simulink model "bldc_with_svpwm"  (R2022a)
settings: Solver=FixedStepDiscrete  StartTime=0.0  StopTime=1  RelTol=1e-3
undefined symbols (not defined in the file): Ts, Vdc
libraries: simulink x5, slpidlib x3, spsDCVoltageSourceLib x1, spsPermanentMagnetSynchronousMachineLib x1, spsUniversalBridgeLib x1, spspowerguiLib x1
(part 1 of 2)
settings Model: Creator=XieXW  LastModifiedBy=XieXW

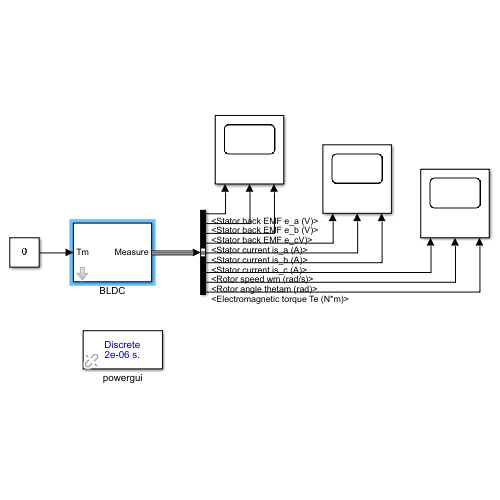
[thumbnail: Simulink's stored preview of the top-level diagram]
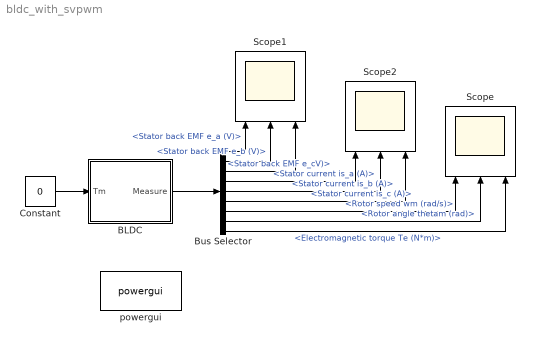
== system bldc_with_svpwm ==
  BLDC : Subsystem  mask{Va=0, Vb=0, Vc=0, t0=0}
      mask prompts: Va "A相电压"; Vb "B相电压"; Vc "C相电压"; t0 "初始角度t0"
      mask DialogControl ParameterGroupVar Prompt: 参数
  Bus Selector : BusSelector  OutputSignals=Stator back EMF e_a (V),Stator back EMF e_b (V),Stator back EMF e_cV),Stator current is_a (A),Stator current is_b (A),Stator current is_c (A),Rotor speed wm (rad/s),Rotor angle thetam (rad),Electromagnetic torque Te (N*m)
  Constant : Constant  Value=0
  Scope : Scope  NumInputPorts=3
  Scope1 : Scope  NumInputPorts=3
  Scope2 : Scope  NumInputPorts=3
  powergui : spspowerguiLib/powergui  Priority=1  SimulationMode=Discrete  SampleTime=2e-6  frequency=60  Iterations=50  frequencyindice=0  Pbase=100e6  ErrMax=1e-4  UnitsV=kV  UnitsW=MW  buscounter=0  FunctionMessages=off  echomessages=off  EnableUseOfTLC=off  CurrentSourceSwitches=off  DisableSnubberDevices=off  DisableRonSwitches=off  DisableVfSwitches=off  DisplayEquations=off  AutomaticDiscreteSolvers=off  SolverType=Tustin/Backward Euler (TBE)  Interpol=off  ExternalGateDelay=off  methode=off  Ts=100  x0status=blocks  SPID=on  SwTol=0  HookPort=off  NonlinearTolerance=1e-4  nMaxIteration=100  ContinueOnMaxIteration=off  RestoreLinks=warning  ResistiveCurrentMeasurement=off  Frange=[0:2:500]  Ylog=off  Xlog=on  ShowGrid=off  save=off  variable=ZData  structure=0  ZoomFFT=off  StartTime=0.0  cycles=1  DisplayStyle=1  fundamental=60  FreqAxis=off  MaxFrequency=1000  frequencyindicesteady=1  RmsSteady=1  display=off
  wires:
  BLDC/1(Measure) -> Bus Selector/1
  Constant/1 -> BLDC/1(Tm)
  Bus Selector/7 -> Scope/1  "<Rotor speed wm (rad/s)>"
  Bus Selector/8 -> Scope/2  "<Rotor angle thetam (rad)>"
  Bus Selector/9 -> Scope/3  "<Electromagnetic torque Te (N*m)>"
  Bus Selector/1 -> Scope1/1  "<Stator back EMF e_a (V)>"
  Bus Selector/2 -> Scope1/2  "<Stator back EMF e_b (V)>"
  Bus Selector/3 -> Scope1/3  "<Stator back EMF e_cV)>"
  Bus Selector/4 -> Scope2/1  "<Stator current is_a (A)>"
  Bus Selector/5 -> Scope2/2  "<Stator current is_b (A)>"
  Bus Selector/6 -> Scope2/3  "<Stator current is_c (A)>"

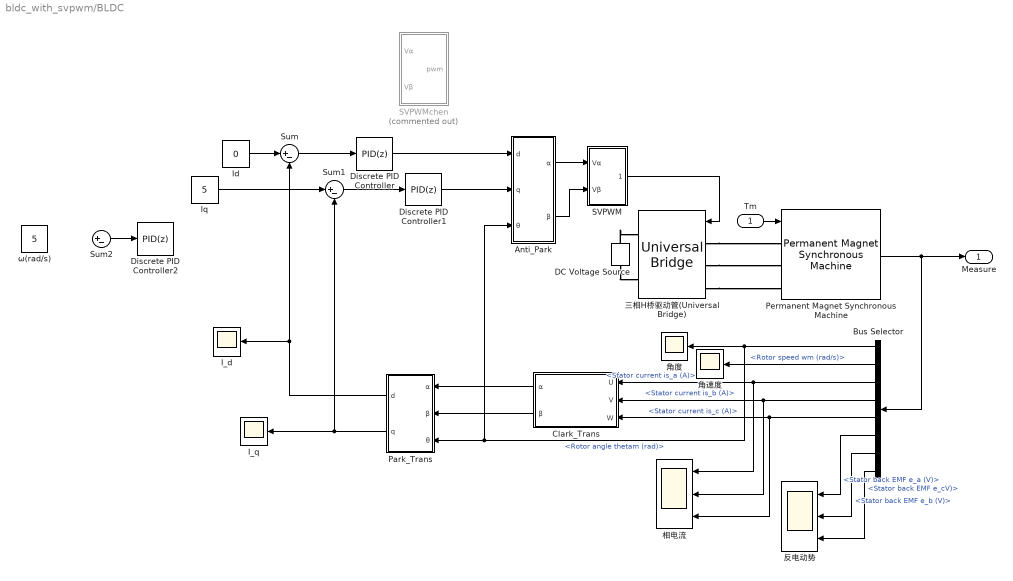
== system bldc_with_svpwm/BLDC ==
  Tm : Inport
  Anti_Park : Subsystem
  Bus Selector : BusSelector  OutputSignals=Rotor angle thetam (rad),Rotor speed wm (rad/s),Stator current is_a (A),Stator current is_b (A),Stator current is_c (A),Stator back EMF e_a (V),Stator back EMF e_b (V),Stator back EMF e_cV)
  Clark_Trans : Subsystem
  DC Voltage Source : spsDCVoltageSourceLib/DC Voltage Source  Amplitude=Vdc  Measurements=None
  Discrete PID Controller : slpidlib/PID Controller  Controller=PID  Form=Parallel  TimeDomain=Discrete-time  UseExternalTs=off  SampleTime=-1  IntegratorMethod=Forward Euler  FilterMethod=Forward Euler  ControllerParametersSource=internal  P=0.5  I=500  UseKiTs=off  D=0  N=100  UseFilter=on  TunerSelectOption=Transfer Function Based (PID Tuner App)  InitialConditionSource=internal  InitialConditionForIntegrator=0  InitialConditionForFilter=0  DifferentiatorICPrevScaledInput=0  ExternalReset=none  TrackingMode=off  Kt=1  LimitOutput=off  SatLimitsSource=internal  UpperSaturationLimit=1  LowerSaturationLimit=-1  LinearizeAsGain=off  AntiWindupMode=none  Kb=1  POutMin=[]  POutMax=[]  IOutMin=[]  IOutMax=[]  DOutMin=[]  DOutMax=[]  NOutMin=[]  NOutMax=[]  SumOutMin=[]  SumOutMax=[]  SaturationOutMin=[]  SaturationOutMax=[]  PParamMin=[]  PParamMax=[]  IParamMin=[]  IParamMax=[]  DParamMin=[]  DParamMax=[]  NParamMin=[]  NParamMax=[]  KbParamMin=[]  KbParamMax=[]  KtParamMin=[]  KtParamMax=[]  KbOutMin=[]  KbOutMax=[]  KtOutMin=[]  KtOutMax=[]  IntegratorOutMin=[]  IntegratorOutMax=[]  FilterOutMin=[]  FilterOutMax=[]  SumI1OutMin=[]  SumI1OutMax=[]  SumI2OutMin=[]  SumI2OutMax=[]  SumI3OutMin=[]  SumI3OutMax=[]  SumI4OutMin=[]  SumI4OutMax=[]  SumDOutMin=[]  SumDOutMax=[]  DifferentiatorOutMin=[]  DifferentiatorOutMax=[]  FilterDiffOutCoefMin=[]  FilterDiffOutCoefMax=[]  ReciprocalOutMin=[]  ReciprocalOutMax=[]  SumDenOutMin=[]  SumDenOutMax=[]  SumNumOutMin=[]  SumNumOutMax=[]  DivideOutMin=[]  DivideOutMax=[]  UdiffTsProdOutMin=[]  UdiffTsProdOutMax=[]  NTsProdOutMin=[]  NTsProdOutMax=[]  UintegralTsProdOutMin=[]  UintegralTsProdOutMax=[]  UngainTsProdOutMin=[]  UngainTsProdOutMax=[]  IntegratorContinuousStateAttributes=''  IntegratorStateMustResolveToSignalObject=off  IntegratorRTWStateStorageClass=Auto  FilterContinuousStateAttributes=''  FilterStateMustResolveToSignalObject=off  FilterRTWStateStorageClass=Auto  ParallelPVariant=InternalParameters  IdealPVariant=Disabled  IVariant=InternalParameters  DVariant=InternalParameters  IntegratorVariant=Discrete  SatVariant=Disabled  AWVariant=Passthrough  PCopyVariant=Disabled  TRVariant=Disabled  FdbkBlocksVariant=Forward  IdealPFdbkVariant=Disabled  SatFdbkVariant=Disabled  DerivativeFilterVariant=ForwardEulerFilter  NVariant=InternalParameters  NCopyVariant=Disabled  FilterICVariant=InternalICsFilter  IntegratorICVariant=InternalICs  ExternalResetVariant=Disabled  TRSumVariant=Passthrough  SumFdbkVariant=Disabled  SumVariant=Sum_PID  TsampFilterVariant=InternalTs  TsampNgainVariant=Passthrough  TsampIntegralVariant=Passthrough  ExternalSaturationOutDataTypeStr=Inherit: Same as second input  aMode=0
  Discrete PID Controller1 : slpidlib/PID Controller  Controller=PID  Form=Parallel  TimeDomain=Discrete-time  UseExternalTs=off  SampleTime=-1  IntegratorMethod=Forward Euler  FilterMethod=Forward Euler  ControllerParametersSource=internal  P=0.5  I=500  UseKiTs=off  D=0  N=100  UseFilter=on  TunerSelectOption=Transfer Function Based (PID Tuner App)  InitialConditionSource=internal  InitialConditionForIntegrator=0  InitialConditionForFilter=0  DifferentiatorICPrevScaledInput=0  ExternalReset=none  TrackingMode=off  Kt=1  LimitOutput=off  SatLimitsSource=internal  UpperSaturationLimit=1  LowerSaturationLimit=-1  LinearizeAsGain=off  AntiWindupMode=none  Kb=1  POutMin=[]  POutMax=[]  IOutMin=[]  IOutMax=[]  DOutMin=[]  DOutMax=[]  NOutMin=[]  NOutMax=[]  SumOutMin=[]  SumOutMax=[]  SaturationOutMin=[]  SaturationOutMax=[]  PParamMin=[]  PParamMax=[]  IParamMin=[]  IParamMax=[]  DParamMin=[]  DParamMax=[]  NParamMin=[]  NParamMax=[]  KbParamMin=[]  KbParamMax=[]  KtParamMin=[]  KtParamMax=[]  KbOutMin=[]  KbOutMax=[]  KtOutMin=[]  KtOutMax=[]  IntegratorOutMin=[]  IntegratorOutMax=[]  FilterOutMin=[]  FilterOutMax=[]  SumI1OutMin=[]  SumI1OutMax=[]  SumI2OutMin=[]  SumI2OutMax=[]  SumI3OutMin=[]  SumI3OutMax=[]  SumI4OutMin=[]  SumI4OutMax=[]  SumDOutMin=[]  SumDOutMax=[]  DifferentiatorOutMin=[]  DifferentiatorOutMax=[]  FilterDiffOutCoefMin=[]  FilterDiffOutCoefMax=[]  ReciprocalOutMin=[]  ReciprocalOutMax=[]  SumDenOutMin=[]  SumDenOutMax=[]  SumNumOutMin=[]  SumNumOutMax=[]  DivideOutMin=[]  DivideOutMax=[]  UdiffTsProdOutMin=[]  UdiffTsProdOutMax=[]  NTsProdOutMin=[]  NTsProdOutMax=[]  UintegralTsProdOutMin=[]  UintegralTsProdOutMax=[]  UngainTsProdOutMin=[]  UngainTsProdOutMax=[]  IntegratorContinuousStateAttributes=''  IntegratorStateMustResolveToSignalObject=off  IntegratorRTWStateStorageClass=Auto  FilterContinuousStateAttributes=''  FilterStateMustResolveToSignalObject=off  FilterRTWStateStorageClass=Auto  ParallelPVariant=InternalParameters  IdealPVariant=Disabled  IVariant=InternalParameters  DVariant=InternalParameters  IntegratorVariant=Discrete  SatVariant=Disabled  AWVariant=Passthrough  PCopyVariant=Disabled  TRVariant=Disabled  FdbkBlocksVariant=Forward  IdealPFdbkVariant=Disabled  SatFdbkVariant=Disabled  DerivativeFilterVariant=ForwardEulerFilter  NVariant=InternalParameters  NCopyVariant=Disabled  FilterICVariant=InternalICsFilter  IntegratorICVariant=InternalICs  ExternalResetVariant=Disabled  TRSumVariant=Passthrough  SumFdbkVariant=Disabled  SumVariant=Sum_PID  TsampFilterVariant=InternalTs  TsampNgainVariant=Passthrough  TsampIntegralVariant=Passthrough  ExternalSaturationOutDataTypeStr=Inherit: Same as second input  aMode=0
  Discrete PID Controller2 : slpidlib/PID Controller  Controller=PID  Form=Parallel  TimeDomain=Discrete-time  UseExternalTs=off  SampleTime=-1  IntegratorMethod=Forward Euler  FilterMethod=Forward Euler  ControllerParametersSource=internal  P=1  I=1  UseKiTs=off  D=0  N=100  UseFilter=on  TunerSelectOption=Transfer Function Based (PID Tuner App)  InitialConditionSource=internal  InitialConditionForIntegrator=0  InitialConditionForFilter=0  DifferentiatorICPrevScaledInput=0  ExternalReset=none  TrackingMode=off  Kt=1  LimitOutput=off  SatLimitsSource=internal  UpperSaturationLimit=inf  LowerSaturationLimit=-inf  LinearizeAsGain=off  AntiWindupMode=none  Kb=1  POutMin=[]  POutMax=[]  IOutMin=[]  IOutMax=[]  DOutMin=[]  DOutMax=[]  NOutMin=[]  NOutMax=[]  SumOutMin=[]  SumOutMax=[]  SaturationOutMin=[]  SaturationOutMax=[]  PParamMin=[]  PParamMax=[]  IParamMin=[]  IParamMax=[]  DParamMin=[]  DParamMax=[]  NParamMin=[]  NParamMax=[]  KbParamMin=[]  KbParamMax=[]  KtParamMin=[]  KtParamMax=[]  KbOutMin=[]  KbOutMax=[]  KtOutMin=[]  KtOutMax=[]  IntegratorOutMin=[]  IntegratorOutMax=[]  FilterOutMin=[]  FilterOutMax=[]  SumI1OutMin=[]  SumI1OutMax=[]  SumI2OutMin=[]  SumI2OutMax=[]  SumI3OutMin=[]  SumI3OutMax=[]  SumI4OutMin=[]  SumI4OutMax=[]  SumDOutMin=[]  SumDOutMax=[]  DifferentiatorOutMin=[]  DifferentiatorOutMax=[]  FilterDiffOutCoefMin=[]  FilterDiffOutCoefMax=[]  ReciprocalOutMin=[]  ReciprocalOutMax=[]  SumDenOutMin=[]  SumDenOutMax=[]  SumNumOutMin=[]  SumNumOutMax=[]  DivideOutMin=[]  DivideOutMax=[]  UdiffTsProdOutMin=[]  UdiffTsProdOutMax=[]  NTsProdOutMin=[]  NTsProdOutMax=[]  UintegralTsProdOutMin=[]  UintegralTsProdOutMax=[]  UngainTsProdOutMin=[]  UngainTsProdOutMax=[]  IntegratorContinuousStateAttributes=''  IntegratorStateMustResolveToSignalObject=off  IntegratorRTWStateStorageClass=Auto  FilterContinuousStateAttributes=''  FilterStateMustResolveToSignalObject=off  FilterRTWStateStorageClass=Auto  ParallelPVariant=InternalParameters  IdealPVariant=Disabled  IVariant=InternalParameters  DVariant=InternalParameters  IntegratorVariant=Discrete  SatVariant=Disabled  AWVariant=Passthrough  PCopyVariant=Disabled  TRVariant=Disabled  FdbkBlocksVariant=Forward  IdealPFdbkVariant=Disabled  SatFdbkVariant=Disabled  DerivativeFilterVariant=ForwardEulerFilter  NVariant=InternalParameters  NCopyVariant=Disabled  FilterICVariant=InternalICsFilter  IntegratorICVariant=InternalICs  ExternalResetVariant=Disabled  TRSumVariant=Passthrough  SumFdbkVariant=Disabled  SumVariant=Sum_PID  TsampFilterVariant=InternalTs  TsampNgainVariant=Passthrough  TsampIntegralVariant=Passthrough  ExternalSaturationOutDataTypeStr=Inherit: Same as second input  aMode=0
  I_d : Scope
  I_q : Scope
  Id : Constant  Value=0
  Iq : Constant  Value=5
  Park_Trans : Subsystem
  Permanent Magnet Synchronous Machine : spsPermanentMagnetSynchronousMachineLib/Permanent Magnet Synchronous Machine  NbPhases=3  FluxDistribution=Trapezoidal  RotorType=Round  MechanicalLoad=Torque Tm  PresetModel=No  ShowDetailedParameters=on  MeasurementBus=off  Resistance=0.0485  Inductance=8.5e-3  dqInductances=[8.5e-3,8.5e-3]  La=0.000395  MachineConstant=Flux linkage established by magnets (V.s)  Flux=0.1194  VoltageCst=25.0071  TorqueCst=0.2388  Flat=120  Mechanical=[0.0027 0.0124924 1 0]  PolePairs=4  InitialConditions=[0,t0, 0,0]  InitialConditions5ph=[0 0 0 0 0 0]  RefAngle=Aligned with phase A axis (original Park)  IterativeDiscreteModel=Trapezoidal non iterative  TsBlock=-1  TsPowergui=0
  SVPWM : Subsystem
  SVPWMchen : Subsystem  Commented=on  mask{Vdc=48, T=1e-4}
      mask prompts: Vdc "直流母线电压Vdc"; T "载波周期T"
      mask DialogControl ParameterGroupVar Prompt: 参数
  Sum : Sum  Inputs=|+-
  Sum1 : Sum  Inputs=|+-
  Sum2 : Sum  Inputs=|+-
  ω(rad/s) : Constant  Value=5
  三相H桥驱动管(Universal Bridge) : spsUniversalBridgeLib/Universal Bridge  Arms=3  SnubberResistance=1e5  SnubberCapacitance=inf  Device=IGBT / Diodes  Ron=1e-3  Lon=0  ForwardVoltages="[  0  0  ]"  ForwardVoltage=0  GTOparameters=[ 10e-6 , 20e-6 ]  IGBTparameters=[ 1e-6 , 2e-6 ]  Measurements=None  Measurements_2=None  converterType=Rectifier
  反电动势 : Scope  NumInputPorts=3
  相电流 : Scope  NumInputPorts=3
  角度 : Scope
  角速度 : Scope
  Measure : Outport
  wires:
  Tm/1 -> Permanent Magnet Synchronous Machine/1
  Permanent Magnet Synchronous Machine/1 -> Bus Selector/1, Measure/1
  Sum/1 -> Discrete PID Controller/1
  Sum1/1 -> Discrete PID Controller1/1
  Id/1 -> Sum/1
  Sum2/1 -> Discrete PID Controller2/1
  Bus Selector/3 -> 相电流/1, Clark_Trans/1(U)  "<Stator current is_a (A)>"
  Bus Selector/4 -> 相电流/2, Clark_Trans/2(V)  "<Stator current is_b (A)>"
  Bus Selector/5 -> 相电流/3, Clark_Trans/3(W)  "<Stator current is_c (A)>"
  Iq/1 -> Sum1/1
  Bus Selector/2 -> 角速度/1  "<Rotor speed wm (rad/s)>"
  Bus Selector/1 -> Park_Trans/3(θ), Anti_Park/3(θ), 角度/1  "<Rotor angle thetam (rad)>"
  Clark_Trans/1(α) -> Park_Trans/1(α)
  Clark_Trans/2(β) -> Park_Trans/2(β)
  Park_Trans/1(d) -> I_d/1, Sum/2
  Park_Trans/2(q) -> I_q/1, Sum1/2
  Discrete PID Controller1/1 -> Anti_Park/2(q)
  Discrete PID Controller/1 -> Anti_Park/1(d)
  Anti_Park/1(α) -> SVPWM/1(Vα)
  Anti_Park/2(β) -> SVPWM/2(Vβ)
  SVPWM/1(pwm) -> 三相H桥驱动管(Universal Bridge)/1
  Bus Selector/6 -> 反电动势/1  "<Stator back EMF e_a (V)>"
  Bus Selector/7 -> 反电动势/2  "<Stator back EMF e_b (V)>"
  Bus Selector/8 -> 反电动势/3  "<Stator back EMF e_cV)>"
  connections:
  三相H桥驱动管(Universal Bridge)/LConn1 -- Permanent Magnet Synchronous Machine/LConn1
  三相H桥驱动管(Universal Bridge)/LConn2 -- Permanent Magnet Synchronous Machine/LConn2
  三相H桥驱动管(Universal Bridge)/LConn3 -- Permanent Magnet Synchronous Machine/LConn3
  DC Voltage Source/RConn1 -- 三相H桥驱动管(Universal Bridge)/RConn1
  DC Voltage Source/LConn1 -- 三相H桥驱动管(Universal Bridge)/RConn2

== system bldc_with_svpwm/BLDC/Anti_Park ==
  d : Inport
  q : Inport  Port=2
  θ : Inport  Port=3
  MATLAB Function1 : MATLAB Function  TreatAsAtomicUnit=on
  MATLAB Function2 : MATLAB Function  TreatAsAtomicUnit=on
  α : Outport
  β : Outport  Port=2
  wires:
  MATLAB Function1/1(alpha) -> α/1
  d/1 -> MATLAB Function2/1(d), MATLAB Function1/1(d)
  q/1 -> MATLAB Function2/2(q), MATLAB Function1/2(q)
  θ/1 -> MATLAB Function2/3(angle), MATLAB Function1/3(angle)
  MATLAB Function2/1(beta) -> β/1

== system bldc_with_svpwm/BLDC/Clark_Trans ==
  U : Inport
  V : Inport  Port=2
  W : Inport  Port=3
  MATLAB Function : MATLAB Function  TreatAsAtomicUnit=on
  MATLAB Function1 : MATLAB Function  TreatAsAtomicUnit=on
  α : Outport
  β : Outport  Port=2
  wires:
  U/1 -> MATLAB Function/1(u)
  V/1 -> MATLAB Function1/1(v), MATLAB Function/2(v)
  W/1 -> MATLAB Function1/2(w), MATLAB Function/3(w)
  MATLAB Function/1(alpha) -> α/1
  MATLAB Function1/1(beta) -> β/1

== system bldc_with_svpwm/BLDC/Park_Trans ==
  α : Inport
  β : Inport  Port=2
  θ : Inport  Port=3
  MATLAB Function : MATLAB Function  TreatAsAtomicUnit=on
  MATLAB Function1 : MATLAB Function  TreatAsAtomicUnit=on
  d : Outport
  q : Outport  Port=2
  wires:
  α/1 -> MATLAB Function/1(alpha), MATLAB Function1/1(alpha)
  MATLAB Function1/1(d) -> d/1
  β/1 -> MATLAB Function/2(beta), MATLAB Function1/2(beta)
  MATLAB Function/1(q) -> q/1
  θ/1 -> MATLAB Function/3(angle), MATLAB Function1/3(angle)

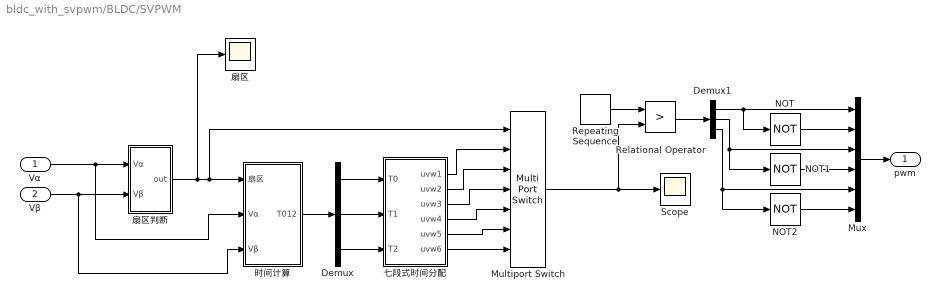
== system bldc_with_svpwm/BLDC/SVPWM ==
  Vα : Inport
  Vβ : Inport  Port=2
  Demux : Demux  Outputs=3
  Demux1 : Demux  Outputs=3
  Multiport Switch : MultiPortSwitch  Inputs=6  SaturateOnIntegerOverflow=off  InputSameDT=off
  Mux : Mux  Inputs=6
  NOT : Logic  Operator=NOT  IconShape=distinctive  AllPortsSameDT=off  OutDataTypeStr=boolean
  NOT1 : Logic  Operator=NOT  IconShape=distinctive  AllPortsSameDT=off  OutDataTypeStr=boolean
  NOT2 : Logic  Operator=NOT  IconShape=distinctive  AllPortsSameDT=off  OutDataTypeStr=boolean
  Relational Operator : RelationalOperator  Operator=>  OutDataTypeStr=boolean  RndMeth=Simplest  InputSameDT=off
  Repeating Sequence : simulink/Sources/Repeating Sequence  rep_seq_t=[0 Ts/2 Ts]  rep_seq_y=[0 1 0]
  Scope : Scope
  七段式时间分配 : Subsystem
  扇区 : Scope
  扇区判断 : Subsystem
  时间计算 : Subsystem
  pwm : Outport
  wires:
  七段式时间分配/6(uvw6) -> Multiport Switch/7
  Demux1/3 -> NOT2/1, Mux/5
  七段式时间分配/5(uvw5) -> Multiport Switch/6
  Demux1/2 -> NOT1/1, Mux/3
  Relational Operator/1 -> Demux1/1
  Demux/1 -> 七段式时间分配/1(T0)
  扇区判断/1(out) -> Multiport Switch/1, 时间计算/1(扇区), 扇区/1
  七段式时间分配/2(uvw2) -> Multiport Switch/3
  Vα/1 -> 时间计算/2(Vα), 扇区判断/1(Vα)
  Vβ/1 -> 时间计算/3(Vβ), 扇区判断/2(Vβ)
  七段式时间分配/1(uvw1) -> Multiport Switch/2
  时间计算/1(T012) -> Demux/1
  七段式时间分配/4(uvw4) -> Multiport Switch/5
  Demux/2 -> 七段式时间分配/2(T1)
  Multiport Switch/1 -> Relational Operator/2, Scope/1
  七段式时间分配/3(uvw3) -> Multiport Switch/4
  Demux/3 -> 七段式时间分配/3(T2)
  Repeating Sequence/1 -> Relational Operator/1
  Demux1/1 -> Mux/1, NOT/1
  NOT2/1 -> Mux/6
  NOT1/1 -> Mux/4
  NOT/1 -> Mux/2
  Mux/1 -> pwm/1

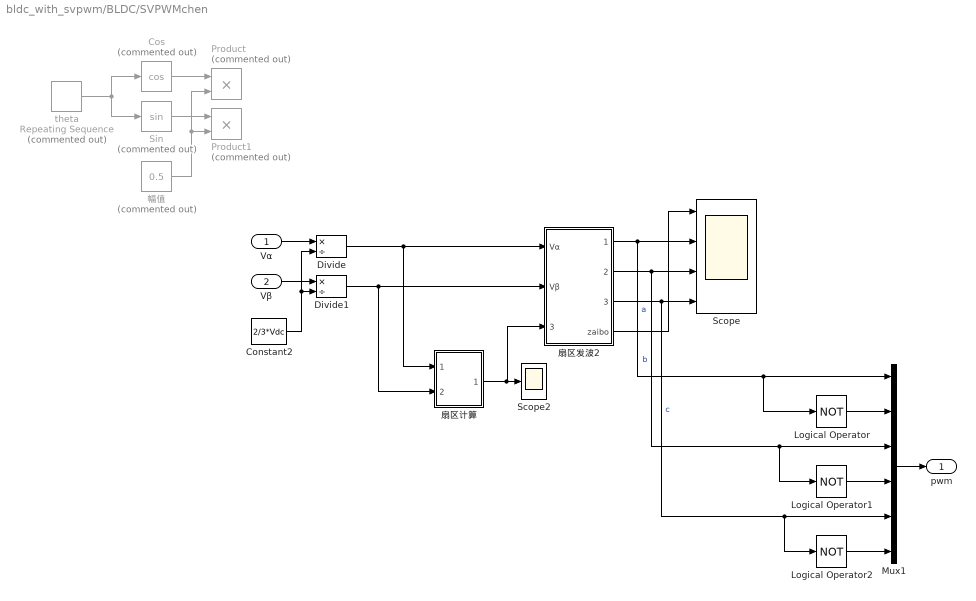
== system bldc_with_svpwm/BLDC/SVPWMchen ==
  Vα : Inport
  Vβ : Inport  Port=2
  Constant2 : Constant  Value=2/3*Vdc
  Cos : Trigonometry  Commented=on  Operator=cos
  Divide : Product  Inputs=*/
  Divide1 : Product  Inputs=*/
  Logical Operator : Logic  Operator=NOT  AllPortsSameDT=off  OutDataTypeStr=boolean
  Logical Operator1 : Logic  Operator=NOT  AllPortsSameDT=off  OutDataTypeStr=boolean
  Logical Operator2 : Logic  Operator=NOT  AllPortsSameDT=off  OutDataTypeStr=boolean
  Mux1 : Mux  Inputs=6
  Product : Product  Commented=on
  Product1 : Product  Commented=on
  Scope : Scope  NumInputPorts=4
  Scope2 : Scope
  Sin : Trigonometry  Commented=on
  theta : simulink/Sources/Repeating Sequence  Commented=on  rep_seq_t=[0 0.002]*pi  rep_seq_y=[0 2]*pi
  幅值 : Constant  Commented=on  Value=0.5
  扇区发波2 : Subsystem  mask{T=T}
      mask prompts: T "载波周期T"
      mask DialogControl ParameterGroupVar Prompt: 参数
  扇区计算 : Subsystem
  pwm : Outport  VectorParamsAs1DForOutWhenUnconnected=off
  wires:
  theta/1 -> Sin/1, Cos/1
  Cos/1 -> Product/1
  Divide1/1 -> 扇区计算/2(Vβ(sin)), 扇区发波2/2(Vβ)
  Divide/1 -> 扇区计算/1(Vα(cos)), 扇区发波2/1(Vα)
  扇区计算/1(Out1) -> 扇区发波2/3(扇区选择), Scope2/1
  幅值/1 -> Product/2, Product1/2
  Sin/1 -> Product1/1
  扇区发波2/4(zaibo) -> Scope/1
  Constant2/1 -> Divide/2, Divide1/2
  Vβ/1 -> Divide1/1
  Vα/1 -> Divide/1
  Logical Operator1/1 -> Mux1/4
  Mux1/1 -> pwm/1
  Logical Operator2/1 -> Mux1/6
  扇区发波2/3(pwm_c) -> Logical Operator2/1, Mux1/5, Scope/4  "c"
  Logical Operator/1 -> Mux1/2
  扇区发波2/1(pwm_a) -> Logical Operator/1, Mux1/1, Scope/2  "a"
  扇区发波2/2(pwm_b) -> Logical Operator1/1, Mux1/3, Scope/3  "b"

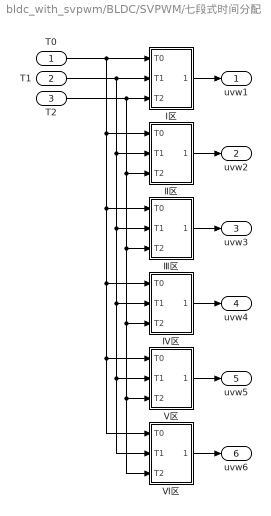
== system bldc_with_svpwm/BLDC/SVPWM/七段式时间分配 ==
  T0 : Inport
  T1 : Inport  Port=2
  T2 : Inport  Port=3
  Ⅰ区 : Subsystem
  Ⅱ区 : Subsystem
  Ⅲ区 : Subsystem
  Ⅳ区 : Subsystem
  Ⅴ区 : Subsystem
  Ⅵ区 : Subsystem
  uvw1 : Outport
  uvw2 : Outport  Port=2
  uvw3 : Outport  Port=3
  uvw4 : Outport  Port=4
  uvw5 : Outport  Port=5
  uvw6 : Outport  Port=6
  wires:
  Ⅱ区/1(uvw2) -> uvw2/1
  T1/1 -> Ⅵ区/2(T1), Ⅴ区/2(T1), Ⅳ区/2(T1), Ⅲ区/2(T1), Ⅱ区/2(T1), Ⅰ区/2(T1)
  Ⅰ区/1(uvw1) -> uvw1/1
  T2/1 -> Ⅵ区/3(T2), Ⅴ区/3(T2), Ⅳ区/3(T2), Ⅲ区/3(T2), Ⅱ区/3(T2), Ⅰ区/3(T2)
  Ⅳ区/1(uvw4) -> uvw4/1
  T0/1 -> Ⅱ区/1(T0), Ⅵ区/1(T0), Ⅴ区/1(T0), Ⅳ区/1(T0), Ⅲ区/1(T0), Ⅰ区/1(T0)
  Ⅵ区/1(uvw6) -> uvw6/1
  Ⅲ区/1(uvw3) -> uvw3/1
  Ⅴ区/1(uvw5) -> uvw5/1

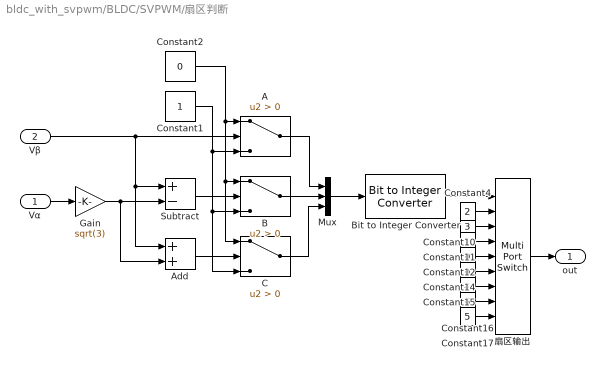
== system bldc_with_svpwm/BLDC/SVPWM/扇区判断 ==
  Vα : Inport
  Vβ : Inport  Port=2
  A : Switch  Criteria=u2 > Threshold  SaturateOnIntegerOverflow=off  InputSameDT=off
  Add : Sum
  B : Switch  Criteria=u2 > Threshold  SaturateOnIntegerOverflow=off  InputSameDT=off
  Bit to Integer Converter : simulink/Logic and Bit Operations/Bit to Integer Converter  nbits=3  bitOrder=MSB first  signedOutputValues=Unsigned  outDtype=Inherit via internal rule  outDtypeSigned=Inherit via internal rule
      settings: SourceProductBaseCode=SL
  C : Switch  Criteria=u2 > Threshold  SaturateOnIntegerOverflow=off  InputSameDT=off
  Constant1 : Constant
  Constant10 : Constant  Value=3
  Constant11 : Constant
  Constant12 : Constant  Value=0
  Constant14 : Constant  Value=0
  Constant15 : Constant  Value=4
  Constant16 : Constant  Value=6
  Constant17 : Constant  Value=5
  Constant2 : Constant  Value=0
  Constant4 : Constant  Value=2
  Gain : Gain  Gain=sqrt(3)
  Mux : Mux  Inputs=3
  Subtract : Sum  Inputs=+-
  扇区输出 : MultiPortSwitch  DataPortOrder=Zero-based contiguous  Inputs=8  zeroidx=on  SaturateOnIntegerOverflow=off  InputSameDT=off
  out : Outport
  wires:
  A/1 -> Mux/1
  Vβ/1 -> A/2, Add/1, Subtract/1
  Mux/1 -> Bit to Integer Converter/1
  Subtract/1 -> B/2
  B/1 -> Mux/2
  Constant2/1 -> C/1, B/1, A/1
  Gain/1 -> Add/2, Subtract/2
  Constant1/1 -> C/3, B/3, A/3
  C/1 -> Mux/3
  Add/1 -> C/2
  Vα/1 -> Gain/1
  扇区输出/1 -> out/1
  Bit to Integer Converter/1 -> 扇区输出/1
  Constant4/1 -> 扇区输出/2
  Constant10/1 -> 扇区输出/3
  Constant11/1 -> 扇区输出/4
  Constant12/1 -> 扇区输出/5
  Constant14/1 -> 扇区输出/6
  Constant15/1 -> 扇区输出/7
  Constant16/1 -> 扇区输出/8
  Constant17/1 -> 扇区输出/9

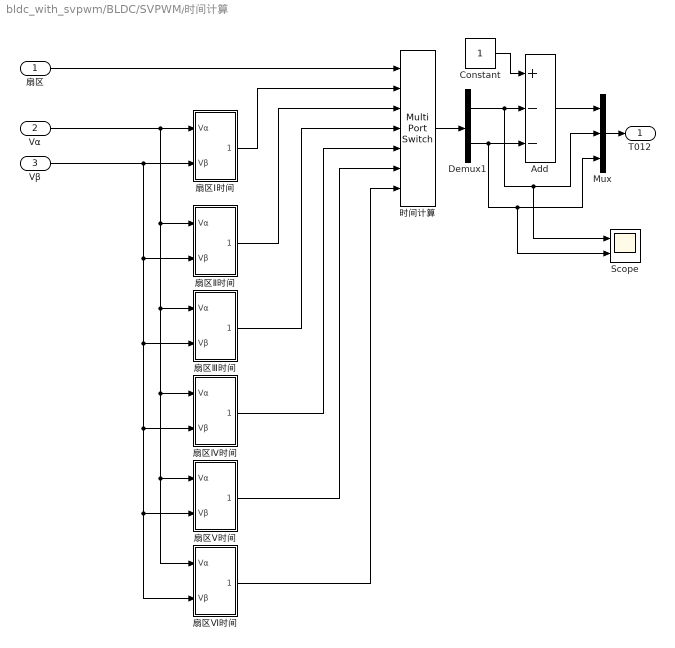
== system bldc_with_svpwm/BLDC/SVPWM/时间计算 ==
  扇区 : Inport
  Vα : Inport  Port=2
  Vβ : Inport  Port=3
  Add : Sum  Inputs=+--
  Constant : Constant
  Demux1 : Demux  Outputs=2
  Mux : Mux  Inputs=3
  Scope : Scope  NumInputPorts=2
  扇区Ⅰ时间 : Subsystem
  扇区Ⅱ时间 : Subsystem
  扇区Ⅲ时间 : Subsystem
  扇区Ⅳ时间 : Subsystem
  扇区Ⅴ时间 : Subsystem
  扇区Ⅵ时间 : Subsystem
  时间计算 : MultiPortSwitch  Inputs=6  SaturateOnIntegerOverflow=off  InputSameDT=off
  T012 : Outport
  wires:
  Vα/1 -> 扇区Ⅵ时间/1(Vα), 扇区Ⅴ时间/1(Vα), 扇区Ⅳ时间/1(Vα), 扇区Ⅲ时间/1(Vα), 扇区Ⅱ时间/1(Vα), 扇区Ⅰ时间/1(Vα)
  时间计算/1 -> Demux1/1
  Demux1/1 -> Scope/1, Mux/2, Add/2
  Add/1 -> Mux/1
  Demux1/2 -> Scope/2, Mux/3, Add/3
  Vβ/1 -> 扇区Ⅵ时间/2(Vβ), 扇区Ⅴ时间/2(Vβ), 扇区Ⅳ时间/2(Vβ), 扇区Ⅲ时间/2(Vβ), 扇区Ⅱ时间/2(Vβ), 扇区Ⅰ时间/2(Vβ)
  Constant/1 -> Add/1
  扇区Ⅰ时间/1(Tout1) -> 时间计算/2
  扇区Ⅴ时间/1(Tout5) -> 时间计算/6
  扇区Ⅳ时间/1(Tout4) -> 时间计算/5
  扇区Ⅱ时间/1(Tout2) -> 时间计算/3
  Mux/1 -> T012/1
  扇区Ⅵ时间/1(Tout6) -> 时间计算/7
  扇区Ⅲ时间/1(Tout3) -> 时间计算/4
  扇区/1 -> 时间计算/1

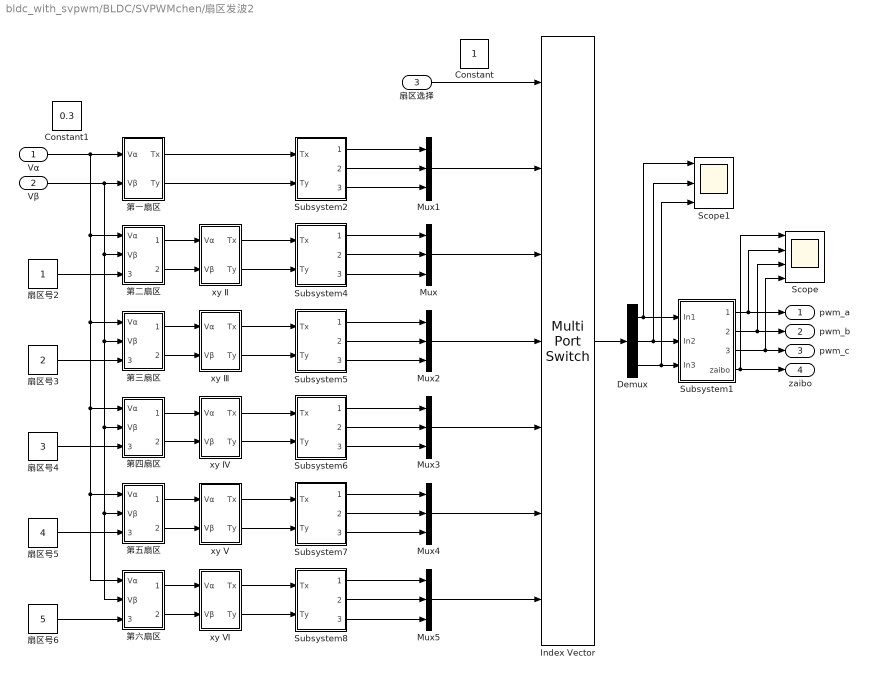
== system bldc_with_svpwm/BLDC/SVPWMchen/扇区发波2 ==
  Vα : Inport
  Vβ : Inport  Port=2
  扇区选择 : Inport  Port=3
  Constant : Constant
  Constant1 : Constant  Value=0.3
  Demux : Demux  Outputs=[1 1 1]
  Index Vector : MultiPortSwitch  Inputs=6  SaturateOnIntegerOverflow=off  InputSameDT=off
  Mux : Mux  Inputs=3
  Mux1 : Mux  Inputs=3
  Mux{2..5} (4 alike) : Mux  Inputs=[1 1 1]
  Scope : Scope  NumInputPorts=4
  Scope1 : Scope  NumInputPorts=3
  Subsystem1 : Subsystem
  Subsystem2 : Subsystem
  Subsystem4 : Subsystem
  Subsystem5 : Subsystem
  Subsystem6 : Subsystem
  Subsystem7 : Subsystem
  Subsystem8 : Subsystem
  xy Ⅱ : Subsystem
  xy Ⅲ : Subsystem
  xy Ⅳ : Subsystem
  xy Ⅴ : Subsystem
  xy Ⅵ : Subsystem
  扇区号2 : Constant
  扇区号3 : Constant  Value=2
  扇区号4 : Constant  Value=3
  扇区号5 : Constant  Value=4
  扇区号6 : Constant  Value=5
  第一扇区 : Subsystem
  第三扇区 : Subsystem
  第二扇区 : Subsystem
  第五扇区 : Subsystem
  第六扇区 : Subsystem
  第四扇区 : Subsystem
  pwm_a : Outport
  pwm_b : Outport  Port=2
  pwm_c : Outport  Port=3
  zaibo : Outport  Port=4
  wires:
  扇区号2/1 -> 第二扇区/3(扇区)
  第二扇区/1(Vα') -> xy Ⅱ/1(Vα)
  第二扇区/2(Vβ') -> xy Ⅱ/2(Vβ)
  Subsystem1/2(pwm_b) -> Scope/3, pwm_b/1
  Subsystem1/1(pwm_a) -> Scope/2, pwm_a/1
  Subsystem1/3(pwm_c) -> Scope/4, pwm_c/1
  Subsystem1/4(zaibo) -> Scope/1, zaibo/1
  Mux1/1 -> Index Vector/2
  Mux/1 -> Index Vector/3
  Demux/1 -> Scope1/1, Subsystem1/1(In1)
  Demux/3 -> Scope1/3, Subsystem1/3(In3)
  第三扇区/2(Vβ') -> xy Ⅲ/2(Vβ)
  第三扇区/1(Vα') -> xy Ⅲ/1(Vα)
  扇区号3/1 -> 第三扇区/3(扇区)
  Mux2/1 -> Index Vector/4
  Mux3/1 -> Index Vector/5
  第四扇区/1(Vα') -> xy Ⅳ/1(Vα)
  第四扇区/2(Vβ') -> xy Ⅳ/2(Vβ)
  扇区号4/1 -> 第四扇区/3(扇区)
  第五扇区/2(Vβ') -> xy Ⅴ/2(Vβ)
  第五扇区/1(Vα') -> xy Ⅴ/1(Vα)
  扇区号5/1 -> 第五扇区/3(扇区)
  扇区号6/1 -> 第六扇区/3(扇区)
  第六扇区/1(Vα') -> xy Ⅵ/1(Vα)
  第六扇区/2(Vβ') -> xy Ⅵ/2(Vβ)
  Index Vector/1 -> Demux/1
  Mux4/1 -> Index Vector/6
  Mux5/1 -> Index Vector/7
  第一扇区/1(Tx) -> Subsystem2/1(Tx)
  第一扇区/2(Ty) -> Subsystem2/2(Ty)
  Subsystem2/1(pwm_a) -> Mux1/1
  Subsystem2/2(pwm_b) -> Mux1/2
  Subsystem2/3(pwm_c) -> Mux1/3
  xy Ⅱ/1(Tx) -> Subsystem4/1(Tx)
  xy Ⅱ/2(Ty) -> Subsystem4/2(Ty)
  Subsystem4/1(pwm_a) -> Mux/1
  Subsystem4/2(pwm_b) -> Mux/2
  Subsystem4/3(pwm_c) -> Mux/3
  Demux/2 -> Scope1/2, Subsystem1/2(In2)
  xy Ⅲ/1(Tx) -> Subsystem5/1(Tx)
  xy Ⅲ/2(Ty) -> Subsystem5/2(Ty)
  Subsystem5/1(pwm_a) -> Mux2/1
  Subsystem5/2(pwm_b) -> Mux2/2
  Subsystem5/3(pwm_c) -> Mux2/3
  Subsystem6/1(pwm_a) -> Mux3/1
  Subsystem6/2(pwm_b) -> Mux3/2
  Subsystem6/3(pwm_c) -> Mux3/3
  xy Ⅳ/1(Tx) -> Subsystem6/1(Tx)
  xy Ⅳ/2(Ty) -> Subsystem6/2(Ty)
  xy Ⅴ/1(Tx) -> Subsystem7/1(Tx)
  xy Ⅴ/2(Ty) -> Subsystem7/2(Ty)
  xy Ⅵ/1(Tx) -> Subsystem8/1(Tx)
  xy Ⅵ/2(Ty) -> Subsystem8/2(Ty)
  Subsystem7/1(pwm_a) -> Mux4/1
  Subsystem7/2(pwm_b) -> Mux4/2
  Subsystem7/3(pwm_c) -> Mux4/3
  Subsystem8/1(pwm_a) -> Mux5/1
  Subsystem8/2(pwm_b) -> Mux5/2
  Subsystem8/3(pwm_c) -> Mux5/3
  扇区选择/1 -> Index Vector/1
  Vα/1 -> 第六扇区/1(Vα), 第五扇区/1(Vα), 第四扇区/1(Vα), 第三扇区/1(Vα), 第二扇区/1(Vα), 第一扇区/1(Vα)
  Vβ/1 -> 第六扇区/2(Vβ), 第五扇区/2(Vβ), 第四扇区/2(Vβ), 第三扇区/2(Vβ), 第二扇区/2(Vβ), 第一扇区/2(Vβ)

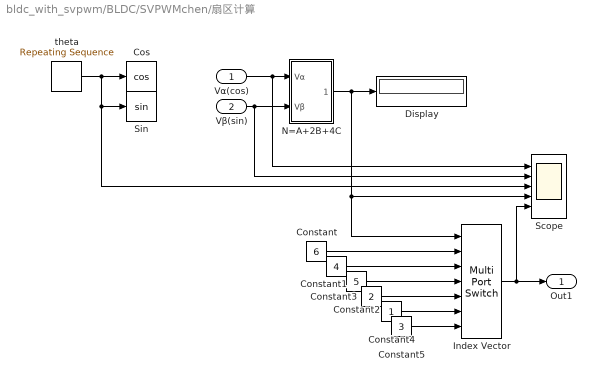
== system bldc_with_svpwm/BLDC/SVPWMchen/扇区计算 ==
  Vα(cos) : Inport
  Vβ(sin) : Inport  Port=2
  Constant : Constant  Value=6
  Constant1 : Constant  Value=4
  Constant2 : Constant  Value=5
  Constant3 : Constant  Value=2
  Constant4 : Constant
  Constant5 : Constant  Value=3
  Cos : Trigonometry  Operator=cos
  Display : Display
  Index Vector : MultiPortSwitch  Inputs=6  SaturateOnIntegerOverflow=off  InputSameDT=off
  N=A+2B+4C : Subsystem
  Scope : Scope  NumInputPorts=5
  Sin : Trigonometry
  theta : simulink/Sources/Repeating Sequence  rep_seq_t=[0 0.01]  rep_seq_y=[0 2]*pi
  Out1 : Outport
  wires:
  N=A+2B+4C/1(Out1) -> Index Vector/1, Scope/4, Display/1
  Index Vector/1 -> Out1/1, Scope/5
  Constant4/1 -> Index Vector/6
  Constant3/1 -> Index Vector/5
  theta/1 -> Scope/3, Sin/1, Cos/1
  Constant1/1 -> Index Vector/3
  Constant5/1 -> Index Vector/7
  Constant2/1 -> Index Vector/4
  Constant/1 -> Index Vector/2
  Vα(cos)/1 -> Scope/1, N=A+2B+4C/1(Vα)
  Vβ(sin)/1 -> Scope/2, N=A+2B+4C/2(Vβ)

== system bldc_with_svpwm/BLDC/SVPWM/七段式时间分配/Ⅰ区 ==
  T0 : Inport
  T1 : Inport  Port=2
  T2 : Inport  Port=3
  Add : Sum  Inputs=+++
  Add1 : Sum
  Gain : Gain  Gain=1/2
  Mux : Mux  Inputs=3
  uvw1 : Outport
  wires:
  Add/1 -> Mux/3
  Gain/1 -> Add/1, Add1/1, Mux/1
  Add1/1 -> Mux/2
  T1/1 -> Add/2, Add1/2
  Mux/1 -> uvw1/1
  T2/1 -> Add/3
  T0/1 -> Gain/1

== system bldc_with_svpwm/BLDC/SVPWM/七段式时间分配/Ⅱ区 ==
  T0 : Inport
  T1 : Inport  Port=2
  T2 : Inport  Port=3
  Add : Sum  Inputs=+++
  Add1 : Sum
  Gain : Gain  Gain=1/2
  Mux : Mux  Inputs=3
  uvw2 : Outport
  wires:
  Mux/1 -> uvw2/1
  T0/1 -> Gain/1
  Gain/1 -> Add/1, Mux/2, Add1/1
  T2/1 -> Add/2, Add1/2
  Add1/1 -> Mux/1
  T1/1 -> Add/3
  Add/1 -> Mux/3

== system bldc_with_svpwm/BLDC/SVPWM/七段式时间分配/Ⅲ区 ==
  T0 : Inport
  T1 : Inport  Port=2
  T2 : Inport  Port=3
  Add : Sum  Inputs=+++
  Add1 : Sum
  Gain : Gain  Gain=1/2
  Mux : Mux  Inputs=3
  uvw3 : Outport
  wires:
  T0/1 -> Gain/1
  T2/1 -> Add/3
  Mux/1 -> uvw3/1
  T1/1 -> Add1/2, Add/2
  Gain/1 -> Mux/2, Add1/1, Add/1
  Add/1 -> Mux/1
  Add1/1 -> Mux/3

== system bldc_with_svpwm/BLDC/SVPWM/七段式时间分配/Ⅳ区 ==
  T0 : Inport
  T1 : Inport  Port=2
  T2 : Inport  Port=3
  Add : Sum  Inputs=+++
  Add1 : Sum
  Gain : Gain  Gain=1/2
  Mux : Mux  Inputs=3
  uvw4 : Outport
  wires:
  Gain/1 -> Add/1, Add1/1, Mux/3
  T0/1 -> Gain/1
  Mux/1 -> uvw4/1
  T2/1 -> Add1/2, Add/2
  T1/1 -> Add/3
  Add/1 -> Mux/1
  Add1/1 -> Mux/2

== system bldc_with_svpwm/BLDC/SVPWM/七段式时间分配/Ⅴ区 ==
  T0 : Inport
  T1 : Inport  Port=2
  T2 : Inport  Port=3
  Add : Sum  Inputs=+++
  Add1 : Sum
  Gain : Gain  Gain=1/2
  Mux : Mux  Inputs=3
  uvw5 : Outport
  wires:
  Gain/1 -> Add/1, Add1/1, Mux/3
  T1/1 -> Add/2, Add1/2
  Mux/1 -> uvw5/1
  T2/1 -> Add/3
  T0/1 -> Gain/1
  Add/1 -> Mux/2
  Add1/1 -> Mux/1

== system bldc_with_svpwm/BLDC/SVPWM/七段式时间分配/Ⅵ区 ==
  T0 : Inport
  T1 : Inport  Port=2
  T2 : Inport  Port=3
  Add : Sum  Inputs=+++
  Add1 : Sum
  Gain : Gain  Gain=1/2
  Mux : Mux  Inputs=3
  uvw6 : Outport
  wires:
  Mux/1 -> uvw6/1
  T0/1 -> Gain/1
  Gain/1 -> Add/1, Add1/2, Mux/1
  T2/1 -> Add/2, Add1/1
  T1/1 -> Add/3
  Add/1 -> Mux/2
  Add1/1 -> Mux/3

== system bldc_with_svpwm/BLDC/SVPWM/时间计算/扇区Ⅰ时间 ==
  Vα : Inport
  Vβ : Inport  Port=2
  Gain : Gain  Gain=1/2
  Mux : Mux  Inputs=2
  Subtract : Sum  Inputs=+-
  sqrt(3)/2 : Gain  Gain=sqrt(3)/2
  Tout1 : Outport
  wires:
  Gain/1 -> Subtract/2
  Vβ/1 -> Mux/2, Gain/1
  Subtract/1 -> Mux/1
  Mux/1 -> Tout1/1
  sqrt(3)/2/1 -> Subtract/1
  Vα/1 -> sqrt(3)/2/1

== system bldc_with_svpwm/BLDC/SVPWM/时间计算/扇区Ⅱ时间 ==
  Vα : Inport
  Vβ : Inport  Port=2
  1/2 : Gain  Gain=1/2
  Gain : Gain  Gain=-1
  Mux : Mux  Inputs=2
  Subtract : Sum
  Subtract1 : Sum
  sqrt(3)/2 : Gain  Gain=sqrt(3)/2
  Tout2 : Outport
  wires:
  Vα/1 -> sqrt(3)/2/1
  Mux/1 -> Tout2/1
  Subtract/1 -> Mux/1
  Vβ/1 -> 1/2/1
  1/2/1 -> Subtract1/2, Subtract/2
  sqrt(3)/2/1 -> Gain/1, Subtract/1
  Subtract1/1 -> Mux/2
  Gain/1 -> Subtract1/1

== system bldc_with_svpwm/BLDC/SVPWM/时间计算/扇区Ⅲ时间 ==
  Vα : Inport
  Vβ : Inport  Port=2
  1/2 : Gain  Gain=1/2
  Gain : Gain  Gain=-1
  Mux : Mux  Inputs=2
  Subtract1 : Sum
  sqrt(3)/2 : Gain  Gain=sqrt(3)/2
  Tout3 : Outport
  wires:
  Vβ/1 -> Mux/1, 1/2/1
  Mux/1 -> Tout3/1
  Vα/1 -> sqrt(3)/2/1
  sqrt(3)/2/1 -> Subtract1/1
  1/2/1 -> Subtract1/2
  Subtract1/1 -> Gain/1
  Gain/1 -> Mux/2

== system bldc_with_svpwm/BLDC/SVPWM/时间计算/扇区Ⅳ时间 ==
  Vα : Inport
  Vβ : Inport  Port=2
  -sqrt(3)/2 : Gain  Gain=-sqrt(3)/2
  1/2 : Gain  Gain=1/2
  Gain : Gain  Gain=-1
  Mux : Mux  Inputs=2
  Subtract : Sum
  Tout4 : Outport
  wires:
  Vα/1 -> -sqrt(3)/2/1
  Mux/1 -> Tout4/1
  Vβ/1 -> Gain/1, 1/2/1
  Gain/1 -> Mux/2
  1/2/1 -> Subtract/2
  -sqrt(3)/2/1 -> Subtract/1
  Subtract/1 -> Mux/1

== system bldc_with_svpwm/BLDC/SVPWM/时间计算/扇区Ⅴ时间 ==
  Vα : Inport
  Vβ : Inport  Port=2
  1/2 : Gain  Gain=1/2
  Gain : Gain  Gain=-1
  Mux : Mux  Inputs=2
  Subtract : Sum
  Subtract1 : Sum  Inputs=+-
  sqrt(3)/2 : Gain  Gain=sqrt(3)/2
  Tout5 : Outport
  wires:
  1/2/1 -> Subtract1/2, Subtract/2
  Vβ/1 -> 1/2/1
  Mux/1 -> Tout5/1
  Vα/1 -> sqrt(3)/2/1
  sqrt(3)/2/1 -> Subtract1/1, Subtract/1
  Subtract/1 -> Gain/1
  Gain/1 -> Mux/1
  Subtract1/1 -> Mux/2

== system bldc_with_svpwm/BLDC/SVPWM/时间计算/扇区Ⅵ时间 ==
  Vα : Inport
  Vβ : Inport  Port=2
  1/2 : Gain  Gain=1/2
  Gain : Gain  Gain=-1
  Mux : Mux  Inputs=2
  Subtract1 : Sum
  sqrt(3)/2 : Gain  Gain=sqrt(3)/2
  Tout6 : Outport
  wires:
  Vα/1 -> sqrt(3)/2/1
  sqrt(3)/2/1 -> Subtract1/1
  Mux/1 -> Tout6/1
  Vβ/1 -> Gain/1, 1/2/1
  1/2/1 -> Subtract1/2
  Subtract1/1 -> Mux/2
  Gain/1 -> Mux/1

== system bldc_with_svpwm/BLDC/SVPWMchen/扇区发波2/Subsystem1 ==
  In1 : Inport
  In2 : Inport  Port=2
  In3 : Inport  Port=3
  Relational Operator : RelationalOperator  Operator=>  OutDataTypeStr=boolean  RndMeth=Simplest  InputSameDT=off
  Relational Operator1 : RelationalOperator  Operator=>  OutDataTypeStr=boolean  RndMeth=Simplest  InputSameDT=off
  Relational Operator2 : RelationalOperator  Operator=>  OutDataTypeStr=boolean  RndMeth=Simplest  InputSameDT=off
  Repeating Sequence : simulink/Sources/Repeating Sequence  rep_seq_t=[0 0.5 1]*T  rep_seq_y=[0 0.5 0]*T
  pwm_a : Outport
  pwm_b : Outport  Port=2
  pwm_c : Outport  Port=3
  zaibo : Outport  Port=4
  wires:
  Repeating Sequence/1 -> Relational Operator1/1, zaibo/1, Relational Operator2/1, Relational Operator/1
  Relational Operator2/1 -> pwm_c/1
  In2/1 -> Relational Operator1/2
  Relational Operator/1 -> pwm_a/1
  In1/1 -> Relational Operator/2
  Relational Operator1/1 -> pwm_b/1
  In3/1 -> Relational Operator2/2

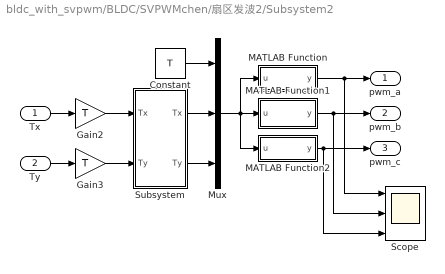
== system bldc_with_svpwm/BLDC/SVPWMchen/扇区发波2/Subsystem2 ==
  Tx : Inport
  Ty : Inport  Port=2
  Constant : Constant  Value=T
  Gain2 : Gain  Gain=T
  Gain3 : Gain  Gain=T
  MATLAB Function : MATLAB Function  TreatAsAtomicUnit=on
  MATLAB Function1 : MATLAB Function  TreatAsAtomicUnit=on
  MATLAB Function2 : MATLAB Function  TreatAsAtomicUnit=on
  Mux : Mux  Inputs=[1 1 1]
  Scope : Scope  NumInputPorts=3
  Subsystem : Subsystem
  pwm_a : Outport
  pwm_b : Outport  Port=2
  pwm_c : Outport  Port=3
  wires:
  Mux/1 -> MATLAB Function1/1(u), MATLAB Function2/1(u), MATLAB Function/1(u)
  MATLAB Function1/1(y) -> pwm_b/1, Scope/2
  Tx/1 -> Gain2/1
  MATLAB Function/1(y) -> pwm_a/1, Scope/1
  MATLAB Function2/1(y) -> pwm_c/1, Scope/3
  Constant/1 -> Mux/1
  Ty/1 -> Gain3/1
  Gain3/1 -> Subsystem/2(Ty)
  Gain2/1 -> Subsystem/1(Tx)
  Subsystem/1("Tx ") -> Mux/2
  Subsystem/2("Ty ") -> Mux/3

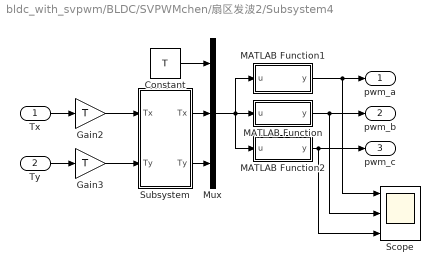
== system bldc_with_svpwm/BLDC/SVPWMchen/扇区发波2/Subsystem4 ==
  Tx : Inport
  Ty : Inport  Port=2
  Constant : Constant  Value=T
  Gain2 : Gain  Gain=T
  Gain3 : Gain  Gain=T
  MATLAB Function : MATLAB Function  TreatAsAtomicUnit=on
  MATLAB Function1 : MATLAB Function  TreatAsAtomicUnit=on
  MATLAB Function2 : MATLAB Function  TreatAsAtomicUnit=on
  Mux : Mux  Inputs=3
  Scope : Scope  NumInputPorts=3
  Subsystem : Subsystem
  pwm_a : Outport
  pwm_b : Outport  Port=2
  pwm_c : Outport  Port=3
  wires:
  Ty/1 -> Gain3/1
  Constant/1 -> Mux/1
  MATLAB Function2/1(y) -> Scope/3, pwm_c/1
  Tx/1 -> Gain2/1
  Mux/1 -> MATLAB Function1/1(u), MATLAB Function/1(u), MATLAB Function2/1(u)
  MATLAB Function/1(y) -> Scope/2, pwm_b/1
  MATLAB Function1/1(y) -> Scope/1, pwm_a/1
  Subsystem/1("Tx ") -> Mux/2
  Subsystem/2("Ty ") -> Mux/3
  Gain2/1 -> Subsystem/1(Tx)
  Gain3/1 -> Subsystem/2(Ty)

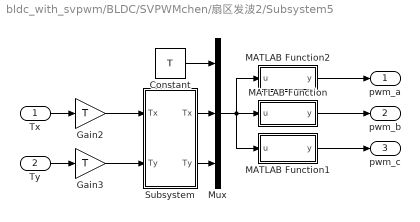
== system bldc_with_svpwm/BLDC/SVPWMchen/扇区发波2/Subsystem5 ==
  Tx : Inport
  Ty : Inport  Port=2
  Constant : Constant  Value=T
  Gain2 : Gain  Gain=T
  Gain3 : Gain  Gain=T
  MATLAB Function : MATLAB Function  TreatAsAtomicUnit=on
  MATLAB Function1 : MATLAB Function  TreatAsAtomicUnit=on
  MATLAB Function2 : MATLAB Function  TreatAsAtomicUnit=on
  Mux : Mux  Inputs=3
  Subsystem : Subsystem
  pwm_a : Outport
  pwm_b : Outport  Port=2
  pwm_c : Outport  Port=3
  wires:
  Tx/1 -> Gain2/1
  Constant/1 -> Mux/1
  Ty/1 -> Gain3/1
  Mux/1 -> MATLAB Function1/1(u), MATLAB Function2/1(u), MATLAB Function/1(u)
  MATLAB Function/1(y) -> pwm_b/1
  MATLAB Function2/1(y) -> pwm_a/1
  MATLAB Function1/1(y) -> pwm_c/1
  Subsystem/1("Tx ") -> Mux/2
  Subsystem/2("Ty ") -> Mux/3
  Gain2/1 -> Subsystem/1(Tx)
  Gain3/1 -> Subsystem/2(Ty)

== system bldc_with_svpwm/BLDC/SVPWMchen/扇区发波2/Subsystem6 ==
  Tx : Inport
  Ty : Inport  Port=2
  Constant : Constant  Value=T
  Gain2 : Gain  Gain=T
  Gain3 : Gain  Gain=T
  MATLAB Function : MATLAB Function  TreatAsAtomicUnit=on
  MATLAB Function1 : MATLAB Function  TreatAsAtomicUnit=on
  MATLAB Function2 : MATLAB Function  TreatAsAtomicUnit=on
  Mux : Mux  Inputs=3
  Subsystem : Subsystem
  pwm_a : Outport
  pwm_b : Outport  Port=2
  pwm_c : Outport  Port=3
  wires:
  MATLAB Function2/1(y) -> pwm_a/1
  Mux/1 -> MATLAB Function/1(u), MATLAB Function1/1(u), MATLAB Function2/1(u)
  Ty/1 -> Gain3/1
  Constant/1 -> Mux/1
  Tx/1 -> Gain2/1
  MATLAB Function1/1(y) -> pwm_b/1
  MATLAB Function/1(y) -> pwm_c/1
  Subsystem/1("Tx ") -> Mux/2
  Subsystem/2("Ty ") -> Mux/3
  Gain2/1 -> Subsystem/1(Tx)
  Gain3/1 -> Subsystem/2(Ty)

== system bldc_with_svpwm/BLDC/SVPWMchen/扇区发波2/Subsystem7 ==
  Tx : Inport
  Ty : Inport  Port=2
  Constant : Constant  Value=T
  Gain2 : Gain  Gain=T
  Gain3 : Gain  Gain=T
  MATLAB Function : MATLAB Function  TreatAsAtomicUnit=on
  MATLAB Function1 : MATLAB Function  TreatAsAtomicUnit=on
  MATLAB Function2 : MATLAB Function  TreatAsAtomicUnit=on
  Mux : Mux  Inputs=3
  Subsystem : Subsystem
  pwm_a : Outport
  pwm_b : Outport  Port=2
  pwm_c : Outport  Port=3
  wires:
  Tx/1 -> Gain2/1
  Constant/1 -> Mux/1
  Ty/1 -> Gain3/1
  Mux/1 -> MATLAB Function/1(u), MATLAB Function1/1(u), MATLAB Function2/1(u)
  MATLAB Function2/1(y) -> pwm_b/1
  MATLAB Function1/1(y) -> pwm_a/1
  MATLAB Function/1(y) -> pwm_c/1
  Gain2/1 -> Subsystem/1(Tx)
  Gain3/1 -> Subsystem/2(Ty)
  Subsystem/1("Tx ") -> Mux/2
  Subsystem/2("Ty ") -> Mux/3

== system bldc_with_svpwm/BLDC/SVPWMchen/扇区发波2/Subsystem8 ==
  Tx : Inport
  Ty : Inport  Port=2
  Constant : Constant  Value=T
  Gain2 : Gain  Gain=T
  Gain3 : Gain  Gain=T
  MATLAB Function : MATLAB Function  TreatAsAtomicUnit=on
  MATLAB Function1 : MATLAB Function  TreatAsAtomicUnit=on
  MATLAB Function2 : MATLAB Function  TreatAsAtomicUnit=on
  Mux : Mux  Inputs=3
  Subsystem : Subsystem
  pwm_a : Outport
  pwm_b : Outport  Port=2
  pwm_c : Outport  Port=3
  wires:
  Ty/1 -> Gain3/1
  Constant/1 -> Mux/1
  Tx/1 -> Gain2/1
  MATLAB Function/1(y) -> pwm_a/1
  MATLAB Function2/1(y) -> pwm_b/1
  MATLAB Function1/1(y) -> pwm_c/1
  Mux/1 -> MATLAB Function/1(u), MATLAB Function2/1(u), MATLAB Function1/1(u)
  Subsystem/1("Tx ") -> Mux/2
  Subsystem/2("Ty ") -> Mux/3
  Gain2/1 -> Subsystem/1(Tx)
  Gain3/1 -> Subsystem/2(Ty)

== system bldc_with_svpwm/BLDC/SVPWMchen/扇区发波2/xy Ⅱ ==
  note: 第一象限的Tx',Ty'转化为
      | 第二象限的Tx,Ty
  Vα : Inport
  Vβ : Inport  Port=2
  Gain4 : Gain  Gain=1/sqrt(3)
  Gain5 : Gain  Gain=2
  Sum1 : Sum  Inputs=|+-
  Tx : Outport
  Ty : Outport  Port=2
  wires:
  Gain4/1 -> Sum1/2, Gain5/1
  Vβ/1 -> Gain4/1
  Vα/1 -> Sum1/1
  Sum1/1 -> Ty/1  "Tx‘"
  Gain5/1 -> Tx/1  "Ty’"

== system bldc_with_svpwm/BLDC/SVPWMchen/扇区发波2/xy Ⅲ ==
  note: 第一扇区的Tx',Ty'转化为
      | 第三扇区的Tx,Ty
  Vα : Inport
  Vβ : Inport  Port=2
  Gain4 : Gain  Gain=1/sqrt(3)
  Gain5 : Gain  Gain=2
  Sum1 : Sum  Inputs=|+-
  Tx : Outport
  Ty : Outport  Port=2
  wires:
  Vα/1 -> Sum1/1
  Vβ/1 -> Gain4/1
  Gain4/1 -> Sum1/2, Gain5/1
  Sum1/1 -> Tx/1  "Tx'"
  Gain5/1 -> Ty/1  "Ty’"

== system bldc_with_svpwm/BLDC/SVPWMchen/扇区发波2/xy Ⅳ ==
  note: 第一扇区的Tx',Ty'转化为
      | 第四扇区的Tx,Ty
  Vα : Inport
  Vβ : Inport  Port=2
  Gain4 : Gain  Gain=1/sqrt(3)
  Gain5 : Gain  Gain=2
  Sum1 : Sum  Inputs=|+-
  Tx : Outport
  Ty : Outport  Port=2
  wires:
  Gain4/1 -> Gain5/1, Sum1/2
  Vβ/1 -> Gain4/1
  Vα/1 -> Sum1/1
  Sum1/1 -> Ty/1  "Tx'"
  Gain5/1 -> Tx/1  "Ty’"

== system bldc_with_svpwm/BLDC/SVPWMchen/扇区发波2/xy Ⅴ ==
  note: 第一扇区的Tx',Ty'转化为
      | 第五扇区的Tx,Ty
  Vα : Inport
  Vβ : Inport  Port=2
  Gain4 : Gain  Gain=1/sqrt(3)
  Gain5 : Gain  Gain=2
  Sum1 : Sum  Inputs=|+-
  Tx : Outport
  Ty : Outport  Port=2
  wires:
  Vα/1 -> Sum1/1
  Vβ/1 -> Gain4/1
  Gain4/1 -> Sum1/2, Gain5/1
  Sum1/1 -> Tx/1  "Tx'"
  Gain5/1 -> Ty/1  "Ty’"

== system bldc_with_svpwm/BLDC/SVPWMchen/扇区发波2/xy Ⅵ ==
  note: 第一扇区的Tx',Ty'转化为
      | 第六扇区的Tx,Ty
  Vα : Inport
  Vβ : Inport  Port=2
  Gain4 : Gain  Gain=1/sqrt(3)
  Gain5 : Gain  Gain=2
  Sum1 : Sum  Inputs=|+-
  Tx : Outport
  Ty : Outport  Port=2
  wires:
  Gain4/1 -> Gain5/1, Sum1/2
  Vβ/1 -> Gain4/1
  Vα/1 -> Sum1/1
  Sum1/1 -> Ty/1  "Tx'"
  Gain5/1 -> Tx/1  "Ty’"

== system bldc_with_svpwm/BLDC/SVPWMchen/扇区发波2/第一扇区 ==
  note: 此处为第二象限的Vα,Vβ
  Vα : Inport
  Vβ : Inport  Port=2
  Gain : Gain  Gain=1/sqrt(3)
  Gain1 : Gain  Gain=2
  Sum : Sum  Inputs=|+-
  Tx : Outport
  Ty : Outport  Port=2
  wires:
  Gain/1 -> Gain1/1, Sum/2
  Gain1/1 -> Ty/1  "Ty"
  Vβ/1 -> Gain/1
  Vα/1 -> Sum/1
  Sum/1 -> Tx/1  "Tx"

== system bldc_with_svpwm/BLDC/SVPWMchen/扇区发波2/第三扇区 ==
  note: 第一象限的Vα,Vβ
  Vα : Inport
  Vβ : Inport  Port=2
  扇区 : Inport  Port=3
  Complex to Magnitude-Angle : ComplexToMagnitudeAngle
  Complex to Real-Imag1 : ComplexToRealImag
  Gain4 : Gain  Gain=-pi/3
  Magnitude-Angle to Complex : MagnitudeAngleToComplex
  Real-Imag to Complex : RealImagToComplex
  Sum1 : Sum  Inputs=|++
  Vα' : Outport
  Vβ' : Outport  Port=2
  wires:
  Vα/1 -> Real-Imag to Complex/1
  Complex to Real-Imag1/2 -> Vβ'/1
  Magnitude-Angle to Complex/1 -> Complex to Real-Imag1/1
  Complex to Real-Imag1/1 -> Vα'/1
  Sum1/1 -> Magnitude-Angle to Complex/2
  Gain4/1 -> Sum1/2
  扇区/1 -> Gain4/1
  Complex to Magnitude-Angle/1 -> Magnitude-Angle to Complex/1
  Vβ/1 -> Real-Imag to Complex/2
  Real-Imag to Complex/1 -> Complex to Magnitude-Angle/1
  Complex to Magnitude-Angle/2 -> Sum1/1

== system bldc_with_svpwm/BLDC/SVPWMchen/扇区发波2/第二扇区 ==
  note: 第一象限的Vα,Vβ
  Vα : Inport
  Vβ : Inport  Port=2
  扇区 : Inport  Port=3
  Complex to Magnitude-Angle : ComplexToMagnitudeAngle
  Complex to Real-Imag1 : ComplexToRealImag
  Gain4 : Gain  Gain=-pi/3
  Magnitude-Angle to Complex : MagnitudeAngleToComplex
  Real-Imag to Complex : RealImagToComplex
  Sum1 : Sum  Inputs=|++
  Vα' : Outport
  Vβ' : Outport  Port=2
  wires:
  Complex to Magnitude-Angle/2 -> Sum1/1
  Real-Imag to Complex/1 -> Complex to Magnitude-Angle/1
  Vβ/1 -> Real-Imag to Complex/2
  Complex to Magnitude-Angle/1 -> Magnitude-Angle to Complex/1
  扇区/1 -> Gain4/1
  Gain4/1 -> Sum1/2
  Sum1/1 -> Magnitude-Angle to Complex/2
  Complex to Real-Imag1/1 -> Vα'/1
  Magnitude-Angle to Complex/1 -> Complex to Real-Imag1/1
  Complex to Real-Imag1/2 -> Vβ'/1
  Vα/1 -> Real-Imag to Complex/1

== system bldc_with_svpwm/BLDC/SVPWMchen/扇区发波2/第五扇区 ==
  note: 第一象限的Vα,Vβ
  Vα : Inport
  Vβ : Inport  Port=2
  扇区 : Inport  Port=3
  Complex to Magnitude-Angle : ComplexToMagnitudeAngle
  Complex to Real-Imag1 : ComplexToRealImag
  Gain4 : Gain  Gain=-pi/3
  Magnitude-Angle to Complex : MagnitudeAngleToComplex
  Real-Imag to Complex : RealImagToComplex
  Sum1 : Sum  Inputs=|++
  Vα' : Outport
  Vβ' : Outport  Port=2
  wires:
  Vα/1 -> Real-Imag to Complex/1
  Complex to Real-Imag1/2 -> Vβ'/1
  Magnitude-Angle to Complex/1 -> Complex to Real-Imag1/1
  Complex to Real-Imag1/1 -> Vα'/1
  Sum1/1 -> Magnitude-Angle to Complex/2
  Gain4/1 -> Sum1/2
  扇区/1 -> Gain4/1
  Complex to Magnitude-Angle/1 -> Magnitude-Angle to Complex/1
  Vβ/1 -> Real-Imag to Complex/2
  Real-Imag to Complex/1 -> Complex to Magnitude-Angle/1
  Complex to Magnitude-Angle/2 -> Sum1/1

== system bldc_with_svpwm/BLDC/SVPWMchen/扇区发波2/第六扇区 ==
  note: 第一象限的Vα,Vβ
  Vα : Inport
  Vβ : Inport  Port=2
  扇区 : Inport  Port=3
  Complex to Magnitude-Angle : ComplexToMagnitudeAngle
  Complex to Real-Imag1 : ComplexToRealImag
  Gain4 : Gain  Gain=-pi/3
  Magnitude-Angle to Complex : MagnitudeAngleToComplex
  Real-Imag to Complex : RealImagToComplex
  Sum1 : Sum  Inputs=|++
  Vα' : Outport
  Vβ' : Outport  Port=2
  wires:
  Complex to Magnitude-Angle/2 -> Sum1/1
  Real-Imag to Complex/1 -> Complex to Magnitude-Angle/1
  Vβ/1 -> Real-Imag to Complex/2
  Complex to Magnitude-Angle/1 -> Magnitude-Angle to Complex/1
  扇区/1 -> Gain4/1
  Gain4/1 -> Sum1/2
  Sum1/1 -> Magnitude-Angle to Complex/2
  Complex to Real-Imag1/1 -> Vα'/1
  Magnitude-Angle to Complex/1 -> Complex to Real-Imag1/1
  Complex to Real-Imag1/2 -> Vβ'/1
  Vα/1 -> Real-Imag to Complex/1

== system bldc_with_svpwm/BLDC/SVPWMchen/扇区发波2/第四扇区 ==
  note: 第一象限的Vα,Vβ
  Vα : Inport
  Vβ : Inport  Port=2
  扇区 : Inport  Port=3
  Complex to Magnitude-Angle : ComplexToMagnitudeAngle
  Complex to Real-Imag1 : ComplexToRealImag
  Gain4 : Gain  Gain=-pi/3
  Magnitude-Angle to Complex : MagnitudeAngleToComplex
  Real-Imag to Complex : RealImagToComplex
  Sum1 : Sum  Inputs=|++
  Vα' : Outport
  Vβ' : Outport  Port=2
  wires:
  Complex to Magnitude-Angle/2 -> Sum1/1
  Real-Imag to Complex/1 -> Complex to Magnitude-Angle/1
  Vβ/1 -> Real-Imag to Complex/2
  Complex to Magnitude-Angle/1 -> Magnitude-Angle to Complex/1
  扇区/1 -> Gain4/1
  Gain4/1 -> Sum1/2
  Sum1/1 -> Magnitude-Angle to Complex/2
  Complex to Real-Imag1/1 -> Vα'/1
  Magnitude-Angle to Complex/1 -> Complex to Real-Imag1/1
  Complex to Real-Imag1/2 -> Vβ'/1
  Vα/1 -> Real-Imag to Complex/1

== system bldc_with_svpwm/BLDC/SVPWMchen/扇区计算/N=A+2B+4C ==
  Vα : Inport
  Vβ : Inport  Port=2
  A : Subsystem
  B : Subsystem
  C : Subsystem
  Gain : Gain
  Gain1 : Gain  Gain=2
  Gain2 : Gain  Gain=4
  Sum : Sum  Inputs=|+++
  Out1 : Outport
  wires:
  Vβ/1 -> C/1(Vβ), B/2(Vβ), A/2(Vβ)
  B/1(Out1) -> Gain1/1
  Gain/1 -> Sum/1
  A/1(Out1) -> Gain/1
  Vα/1 -> B/1(Vα), A/1(Vα)
  C/1(Out1) -> Gain2/1
  Gain1/1 -> Sum/2
  Gain2/1 -> Sum/3
  Sum/1 -> Out1/1

== system bldc_with_svpwm/BLDC/SVPWMchen/扇区发波2/Subsystem2/Subsystem ==
  Tx : Inport
  Ty : Inport  Port=2
  Constant1 : Constant  Value=T
  Divide : Product  Inputs=*/
  Divide1 : Product  Inputs=*/
  Gain : Gain  Gain=T
  Gain1 : Gain  Gain=T
  Relational Operator : RelationalOperator  Operator=<=  OutDataTypeStr=boolean  RndMeth=Simplest  InputSameDT=off
  Sum : Sum
  Switch : Switch  Criteria=u2 > Threshold  SaturateOnIntegerOverflow=off  InputSameDT=off
  Switch1 : Switch  Criteria=u2 > Threshold  SaturateOnIntegerOverflow=off  InputSameDT=off
  "Tx " : Outport  VectorParamsAs1DForOutWhenUnconnected=off
  "Ty " : Outport  Port=2  VectorParamsAs1DForOutWhenUnconnected=off
  wires:
  Switch/1 -> "Tx "/1
  Sum/1 -> Relational Operator/1, Divide1/2, Divide/2  "Tx+Ty"
  Tx/1 -> Sum/1, Switch/1, Divide/1  "Tx"
  Relational Operator/1 -> Switch/2, Switch1/2
  Ty/1 -> Sum/2, Divide1/1, Switch1/1
  Divide1/1 -> Gain1/1
  Divide/1 -> Gain/1
  Switch1/1 -> "Ty "/1
  Constant1/1 -> Relational Operator/2
  Gain/1 -> Switch/3
  Gain1/1 -> Switch1/3

== system bldc_with_svpwm/BLDC/SVPWMchen/扇区发波2/Subsystem4/Subsystem ==
  Tx : Inport
  Ty : Inport  Port=2
  Constant1 : Constant  Value=T
  Divide : Product  Inputs=*/
  Divide1 : Product  Inputs=*/
  Gain : Gain  Gain=T
  Gain1 : Gain  Gain=T
  Relational Operator : RelationalOperator  Operator=<=  OutDataTypeStr=boolean  RndMeth=Simplest  InputSameDT=off
  Sum : Sum
  Switch : Switch  Criteria=u2 > Threshold  SaturateOnIntegerOverflow=off  InputSameDT=off
  Switch1 : Switch  Criteria=u2 > Threshold  SaturateOnIntegerOverflow=off  InputSameDT=off
  "Tx " : Outport  VectorParamsAs1DForOutWhenUnconnected=off
  "Ty " : Outport  Port=2  VectorParamsAs1DForOutWhenUnconnected=off
  wires:
  Switch/1 -> "Tx "/1
  Sum/1 -> Relational Operator/1, Divide1/2, Divide/2  "Tx+Ty"
  Tx/1 -> Sum/1, Switch/1, Divide/1  "Tx"
  Relational Operator/1 -> Switch/2, Switch1/2
  Ty/1 -> Sum/2, Divide1/1, Switch1/1
  Divide1/1 -> Gain1/1
  Divide/1 -> Gain/1
  Switch1/1 -> "Ty "/1
  Constant1/1 -> Relational Operator/2
  Gain/1 -> Switch/3
  Gain1/1 -> Switch1/3

== system bldc_with_svpwm/BLDC/SVPWMchen/扇区发波2/Subsystem5/Subsystem ==
  Tx : Inport
  Ty : Inport  Port=2
  Constant1 : Constant  Value=T
  Divide : Product  Inputs=*/
  Divide1 : Product  Inputs=*/
  Gain : Gain  Gain=T
  Gain1 : Gain  Gain=T
  Relational Operator : RelationalOperator  Operator=<=  OutDataTypeStr=boolean  RndMeth=Simplest  InputSameDT=off
  Sum : Sum
  Switch : Switch  Criteria=u2 > Threshold  SaturateOnIntegerOverflow=off  InputSameDT=off
  Switch1 : Switch  Criteria=u2 > Threshold  SaturateOnIntegerOverflow=off  InputSameDT=off
  "Tx " : Outport  VectorParamsAs1DForOutWhenUnconnected=off
  "Ty " : Outport  Port=2  VectorParamsAs1DForOutWhenUnconnected=off
  wires:
  Switch/1 -> "Tx "/1
  Sum/1 -> Relational Operator/1, Divide1/2, Divide/2  "Tx+Ty"
  Tx/1 -> Sum/1, Switch/1, Divide/1  "Tx"
  Relational Operator/1 -> Switch/2, Switch1/2
  Ty/1 -> Sum/2, Divide1/1, Switch1/1
  Divide1/1 -> Gain1/1
  Divide/1 -> Gain/1
  Switch1/1 -> "Ty "/1
  Constant1/1 -> Relational Operator/2
  Gain/1 -> Switch/3
  Gain1/1 -> Switch1/3

== system bldc_with_svpwm/BLDC/SVPWMchen/扇区发波2/Subsystem6/Subsystem ==
  Tx : Inport
  Ty : Inport  Port=2
  Constant1 : Constant  Value=T
  Divide : Product  Inputs=*/
  Divide1 : Product  Inputs=*/
  Gain : Gain  Gain=T
  Gain1 : Gain  Gain=T
  Relational Operator : RelationalOperator  Operator=<=  OutDataTypeStr=boolean  RndMeth=Simplest  InputSameDT=off
  Sum : Sum
  Switch : Switch  Criteria=u2 > Threshold  SaturateOnIntegerOverflow=off  InputSameDT=off
  Switch1 : Switch  Criteria=u2 > Threshold  SaturateOnIntegerOverflow=off  InputSameDT=off
  "Tx " : Outport  VectorParamsAs1DForOutWhenUnconnected=off
  "Ty " : Outport  Port=2  VectorParamsAs1DForOutWhenUnconnected=off
  wires:
  Switch/1 -> "Tx "/1
  Sum/1 -> Relational Operator/1, Divide1/2, Divide/2  "Tx+Ty"
  Tx/1 -> Sum/1, Switch/1, Divide/1  "Tx"
  Relational Operator/1 -> Switch/2, Switch1/2
  Ty/1 -> Sum/2, Divide1/1, Switch1/1
  Divide1/1 -> Gain1/1
  Divide/1 -> Gain/1
  Switch1/1 -> "Ty "/1
  Constant1/1 -> Relational Operator/2
  Gain/1 -> Switch/3
  Gain1/1 -> Switch1/3

== system bldc_with_svpwm/BLDC/SVPWMchen/扇区发波2/Subsystem7/Subsystem ==
  Tx : Inport
  Ty : Inport  Port=2
  Constant1 : Constant  Value=T
  Divide : Product  Inputs=*/
  Divide1 : Product  Inputs=*/
  Gain : Gain  Gain=T
  Gain1 : Gain  Gain=T
  Relational Operator : RelationalOperator  Operator=<=  OutDataTypeStr=boolean  RndMeth=Simplest  InputSameDT=off
  Sum : Sum
  Switch : Switch  Criteria=u2 > Threshold  SaturateOnIntegerOverflow=off  InputSameDT=off
  Switch1 : Switch  Criteria=u2 > Threshold  SaturateOnIntegerOverflow=off  InputSameDT=off
  "Tx " : Outport  VectorParamsAs1DForOutWhenUnconnected=off
  "Ty " : Outport  Port=2  VectorParamsAs1DForOutWhenUnconnected=off
  wires:
  Switch/1 -> "Tx "/1
  Sum/1 -> Relational Operator/1, Divide1/2, Divide/2  "Tx+Ty"
  Tx/1 -> Sum/1, Switch/1, Divide/1  "Tx"
  Relational Operator/1 -> Switch/2, Switch1/2
  Ty/1 -> Sum/2, Divide1/1, Switch1/1
  Divide1/1 -> Gain1/1
  Divide/1 -> Gain/1
  Switch1/1 -> "Ty "/1
  Constant1/1 -> Relational Operator/2
  Gain/1 -> Switch/3
  Gain1/1 -> Switch1/3
